simulink model "Timer_Basics"  (R2025a)
settings: Solver=FixedStepAuto  StartTime=0.0  StopTime=10.0  RelTol=1e-3  EnableMultiTasking=on
libraries: stm32g4xxblockslib x2, simulink x1, stm32f4xxblockslib x1, stm32blockslib x1
settings Model: STM32="{\"HardwareInterrupt\":[{\"ID\":\"Timer_Basics:2\"},{\"ID\":\"Timer_Basics:18\"}],\"TimerBlock\":{\"ID\":\"Timer_Basics:3\"},\"DigitalPortWrite\":{\"ID\":\"Timer_Basics:1\"}}"  Creator=GNKRISHNAN  LastModifiedBy=GNKRISHNAN
settings OptimizationCC: DefaultParameterBehavior=Inlined  EnhancedBackFolding=on  PassReuseOutputArgsAs=Individual arguments  ZeroExternalMemoryAtStartup=off  ZeroInternalMemoryAtStartup=off  MaxStackSize=512  OptimizeBlockOrder=speed  DifferentSizesBufferReuse=on  OptimizationCustomize=off  EfficientTunableParamExpr=on
settings DebuggingCC: ParameterTunabilityLossMsg=error
settings HardwareCC: ProdBitPerPointer=32.0  ProdBitPerSizeT=32.0  ProdBitPerPtrDiffT=32.0  ProdLargestAtomicInteger=Long  ProdLargestAtomicFloat=Double  ProdWordSize=32.0  ProdLongLongMode=on  ProdHWDeviceType=ARM Compatible->ARM Cortex-M
settings SFSimCC: MATLABDynamicMemAlloc=off
settings RTWCC: SystemTargetFile=ert.tlc  HardwareBoard=STM32G4xx Based  TemplateMakefile=ert_default_tmf  Toolchain=GNU Tools for ARM Embedded Processors  Description=Embedded Coder
settings CodeAppCC: ForceParamTrailComments=on  IgnoreCustomStorageClasses=off  OperatorAnnotations=on  SimulinkDataObjDesc=on  SFDataObjDesc=on  InsertBlockDesc=on
settings ERTTargetCC: ExtModeTransport=3.0  ExtModeStaticAllocSize=2048.0  TargetLangStandard=C99 (ISO)  CodeReplacementLibrary=ARM Cortex-M

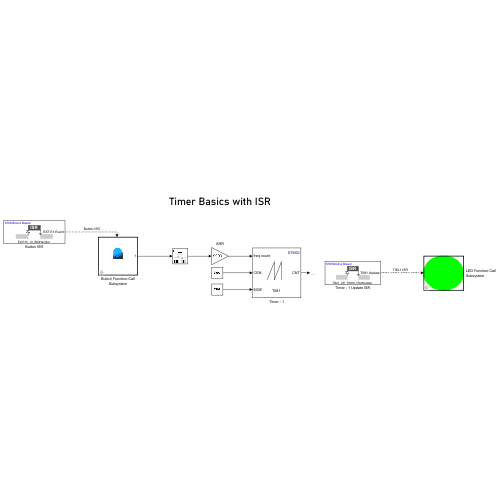
[thumbnail: Simulink's stored preview of the top-level diagram]
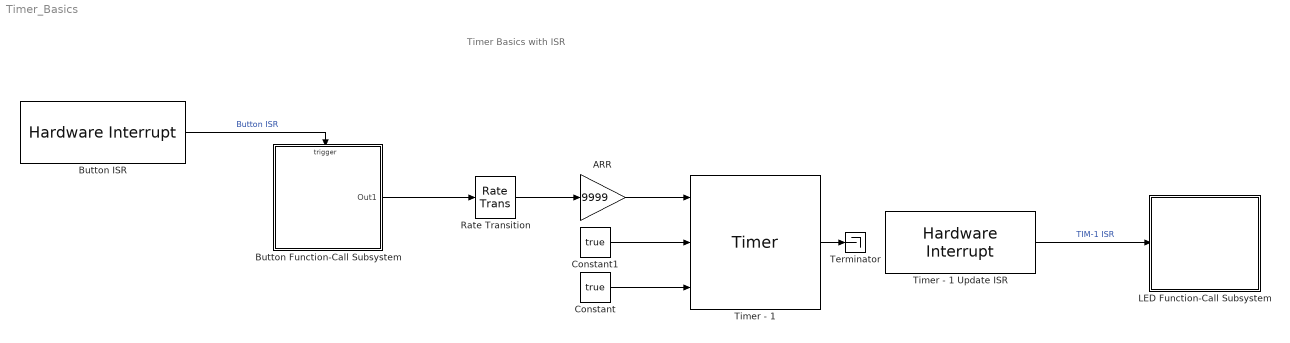
== system Timer_Basics ==
  note: Timer Basics with ISR
  ARR : Gain  Gain=9999
  Button Function-Call Subsystem : Subsystem  TreatAsAtomicUnit=on
      mask Display: image(imread('bttn.png'), [0, 0, 1, 1])
  Button ISR : stm32g4xxblockslib/Hardware Interrupt  ISRGroup=External interrupts (EXTI)  ISRName=EXTI15_10_IRQHandler  ISRNumber=55  EventsList={ 'off', 'EXTI15 Event', '3'; 'off', 'EXTI14 Event', '2'; 'on', 'EXTI13 Event', '1'; 'off', 'EXTI12 Event', '4'; 'off', 'EXTI11 Event', '5'; 'off', 'EXTI10 Event', '6'; 'off', 'Custom event', '7' }  SelectedEvents={'EXTI13 Event'}  TaskPriority=30  DisablePreemption=on  ClearInterruptFlagsAtEndOfEvent=on  InterruptDefinitionFile=$(TARGET_ROOT)/registry/interrupts/STM32F4xxBased_interrupts.xml  HardwareBoard=STM32G4xx Based  EnableSimPort=off
  Constant : Constant  Value=true
  Constant1 : Constant  Value=true
  LED Function-Call Subsystem : Subsystem  TreatAsAtomicUnit=on
      mask Display:
      | color('green');
      | phi = 0:0.1:2*pi;
      | patch(0.5 + 0.3*cos(phi), 0.5 + 0.3*sin(phi), [0 1 0]); % Draws a green circle
  Rate Transition : RateTransition  Deterministic=off  InitialCondition=1
  Terminator : Terminator
  Timer - 1 : stm32blockslib/Timer  TimerModule=TIM1  EnableFrequencyInput=on  EnableCounterInput=on  EnableMainOutputInput=on  SetRCAfterCE=off  OutputDirection=off  OutputMainOutputEnableStatus=off  SampleTime=-1  EnableUpdateEvent=off  EnableCaptureCompare1Event=off  EnableCaptureCompare2Event=off  EnableCaptureCompare3Event=off  EnableCaptureCompare4Event=off  EnableTriggerEvent=off  EnableBreakEvent=off  EnableBreakEvent2=off  EnableCOMGenerationEvent=off  ProcessorFamily=STM32G4
      settings: LibrarySourceBlock=stm32g4xxblockslib/Timer
  Timer - 1 Update ISR : stm32g4xxblockslib/Hardware Interrupt  ISRGroup=Timer (TIM)  ISRName=TIM1_UP_TIM16_IRQHandler  ISRNumber=40  EventsList={ 'on', 'TIM1 Update', '1'; 'off', 'TIM16 Update', '2'; 'off', 'TIM16 CC1', '3'; 'off', 'TIM16 COM', '4'; 'off', 'TIM16 Break', '5'; 'off', 'Custom event', '6' }  SelectedEvents={'TIM1 Update'}  TaskPriority=30  DisablePreemption=on  ClearInterruptFlagsAtEndOfEvent=on  InterruptDefinitionFile=$(TARGET_ROOT)/registry/interrupts/STM32F4xxBased_interrupts.xml  HardwareBoard=STM32G4xx Based  EnableSimPort=off
  wires:
  Constant/1 -> Timer - 1/3
  Constant1/1 -> Timer - 1/2
  Button ISR/1 -> Button Function-Call Subsystem/Trigger  "Button ISR"
  Button Function-Call Subsystem/1(Out1) -> Rate Transition/1
  ARR/1 -> Timer - 1/1
  Timer - 1 Update ISR/1 -> LED Function-Call Subsystem/Trigger  "TIM-1 ISR"
  Rate Transition/1 -> ARR/1
  Timer - 1/1 -> Terminator/1

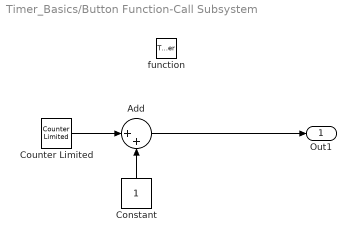
== system Timer_Basics/Button Function-Call Subsystem ==
  function : TriggerPort  TriggerType=function-call  VariantControl=(inherit)
  Add : Sum  Inputs=|++
  Constant : Constant
  Counter Limited : simulink/Sources/Counter Limited  uplimit=2  tsamp=-1
  Out1 : Outport
  wires:
  Add/1 -> Out1/1
  Counter Limited/1 -> Add/1
  Constant/1 -> Add/2

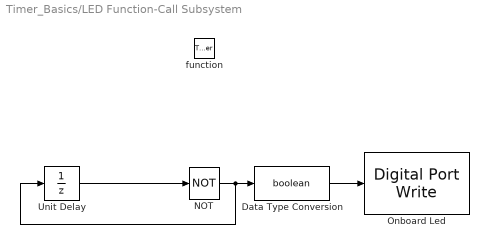
== system Timer_Basics/LED Function-Call Subsystem ==
  function : TriggerPort  TriggerType=function-call  VariantControl=(inherit)
  Data Type Conversion : DataTypeConversion  OutDataTypeStr=boolean  SaturateOnIntegerOverflow=off  RndMeth=Floor
  NOT : Logic  Operator=NOT  IconShape=distinctive  AllPortsSameDT=off  OutDataTypeStr=boolean
  Onboard Led : stm32f4xxblockslib/Digital Port Write  PortName=GPIOA  PinNumber=[5]  ReadOperation=off  IOAsArray=on  EnableSimPort=off  hoistedMaskSrc=ECSoC/ECSimCodegen/Digital Port Write
      settings: LibrarySourceBlock=stm32g4xxblockslib/Digital Port Write
  Unit Delay : UnitDelay  SampleTime=-1  HasFrameUpgradeWarning=on
  wires:
  Unit Delay/1 -> NOT/1
  NOT/1 -> Data Type Conversion/1, Unit Delay/1
  Data Type Conversion/1 -> Onboard Led/1
